simulink model "Diff_equ"  (R2020a)
settings: Solver=VariableStepAuto  StartTime=0.0  StopTime=10.0  RelTol=1e-3
settings Model: Creator=aravi  LastModifiedBy=aravi

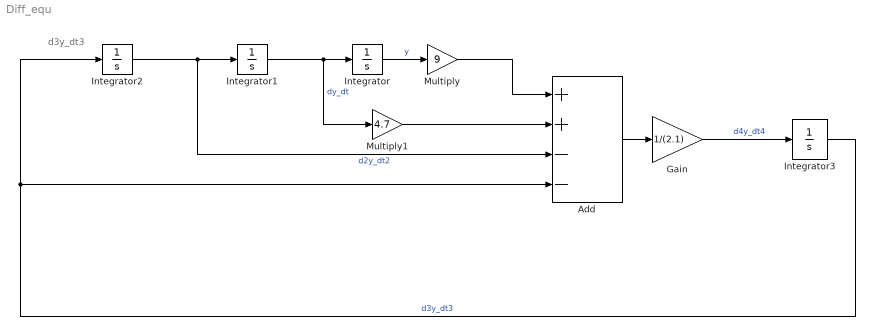
== system Diff_equ ==
  note: d3y_dt3
  Add : Sum  Inputs=++--
  Gain : Gain  Gain=1/(2.1)
  Integrator{,1..3} (4 alike) : Integrator
  Multiply : Gain  Gain=9
  Multiply1 : Gain  Gain=4.7
  wires:
  Integrator/1 -> Multiply/1  "y"
  Multiply/1 -> Add/1
  Integrator1/1 -> Integrator/1, Multiply1/1  "dy_dt"
  Integrator2/1 -> Integrator1/1, Add/3  "d2y_dt2"
  Add/1 -> Gain/1
  Gain/1 -> Integrator3/1  "d4y_dt4"
  Integrator3/1 -> Integrator2/1, Add/4  "d3y_dt3"
  Multiply1/1 -> Add/2
